simulink model "ME416_Autonomy_Model_Rollback2"  (R2025b)
settings: Solver=FixedStepAuto  StartTime=0.0  StopTime=240  RelTol=1e-3  EnableMultiTasking=on
PreLoadFcn:
  | driveparam
values from neighbouring files (symbols this model uses):
  alpha_w = 0.7    [driveparam.m]
  beta = Ts / (Ts + tau)    (= 0.166666666667)    [driveparam.m]
  enable_cmd = 1    [driveparam.m]
  estop_cmd = 0    [driveparam.m]
  K_lqr_w = dlqr(Ad_w, Bd_w, Qw, Rw)    [driveparam.m]
  L = 0.15    [driveparam.m]
  N = 4400    [driveparam.m]
  Nbar_lqr_w = (1 - Ad_w)/Bd_w + K_lqr_w    [driveparam.m]
  r = 0.03    [driveparam.m]
  Ts = 0.01    [driveparam.m]
  v_ref_cmd = 0    [driveparam.m]
  w_ref_cmd = 0.1    [driveparam.m]
undefined symbols (not defined in the file or in its folder): DiscIntNeverNeededParam, dspblkCoreblockFVToolHelper, gcbh
libraries: raspberrypiBasiclib x22, simulink x21, raspberrypiCommlib x19, slpidlib x2
(part 1 of 3)
settings Model: ExtModeTrigDuration=2  Creator=madak  LastModifiedBy=madak
settings SolverCC: PositivePriorityOrder=on  AutoInsertRateTranBlk=on
settings OptimizationCC: EnhancedBackFolding=on  PassReuseOutputArgsAs=Individual arguments  ZeroExternalMemoryAtStartup=off  ZeroInternalMemoryAtStartup=off  MaxStackSize=200000  OptimizeBlockOrder=speed  DifferentSizesBufferReuse=on  OptimizationCustomize=off  EfficientTunableParamExpr=on
settings DebuggingCC: ParameterPrecisionLossMsg=none  ParameterTunabilityLossMsg=error
settings HardwareCC: ProdBitPerLong=64.0  ProdLargestAtomicInteger=LongLong  ProdLargestAtomicFloat=Double  ProdLongLongMode=on  ProdHWDeviceType=ARM Compatible->ARM Cortex-A (64-bit)
settings RTWCC: SystemTargetFile=ert.tlc  HardwareBoard=Raspberry Pi (64bit)  TLCOptions="-aInlineSetEventsForThisBaseRateFcn=TLC_FALSE -aSuppressMultiTaskScheduler=TLC_FALSE  -aRateBasedStepFcn=0"  TemplateMakefile=ert_default_tmf  Toolchain=GNU GCC Embedded Linux  BuildConfiguration=Faster Runs  GPUComputeCapability=3.5  Description=Embedded Coder
settings CodeAppCC: ForceParamTrailComments=on  IgnoreCustomStorageClasses=off  OperatorAnnotations=on  SimulinkDataObjDesc=on  SFDataObjDesc=on  InsertBlockDesc=on
settings ERTTargetCC: ExtModeTransport=2.0  ExtModeStaticAlloc=on  ExtModeMexFile=ext_xcp  ExtModeIntrfLevel=Level2 - Open  InlinedParameterPlacement=Hierarchical  CodeReplacementLibrary=ARM Cortex-A CMSIS  SupportContinuousTime=on  SupportVariableSizeSignals=on

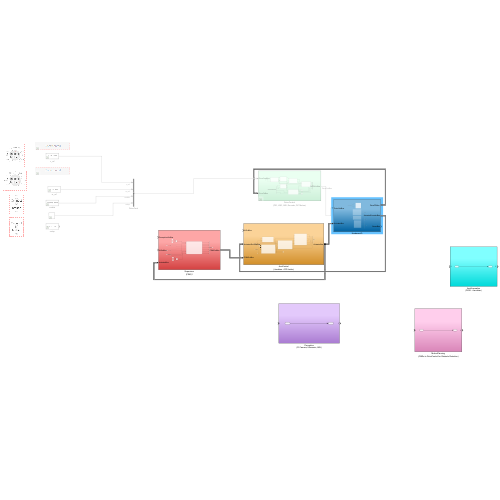
[thumbnail: Simulink's stored preview of the top-level diagram]
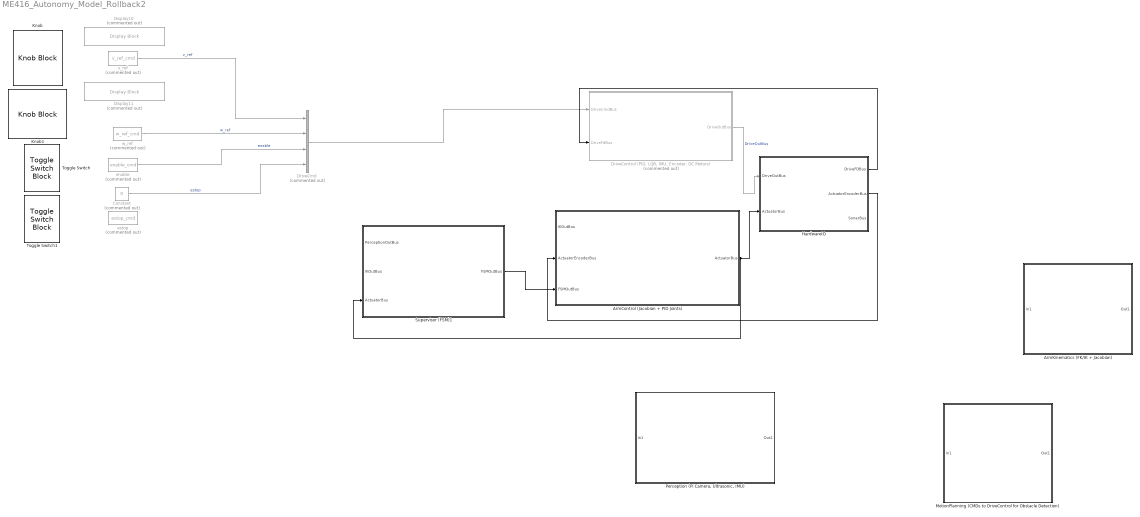
== system ME416_Autonomy_Model_Rollback2 ==
  ArmControl (Jacobian + PID Joints) : Subsystem
  ArmKinematics (FK/IK + Jacobian) : Subsystem
  Constant : Constant  Commented=on  Value=0
  Display10 : DisplayBlock  Commented=on  LabelPosition=Hide  Transparency=1  GridColor=[0.502, 0.502, 0.502]
  Display11 : DisplayBlock  Commented=on  LabelPosition=Hide  Transparency=1  GridColor=[0.502, 0.502, 0.502]
  DriveCmd : BusCreator  Commented=on  Inputs=4
  "DriveControl (PID, LQR, IMU, Encoder, DC Motors)" : Subsystem  Commented=on
  HardwareIO : Subsystem
  Knob : KnobBlock  ScaleMin=-0.5  ScaleMax=0.5  TickInterval=0.1
  Knob1 : KnobBlock  ScaleMin=-1  ScaleMax=1
  MotionPlanning (CMDs to DriveControl for Obstacle Detection) : Subsystem
  "Perception (Pi Camera, Ultrasonic, IMU)" : Subsystem
  Supervisor (FSM)1 : Subsystem
  Toggle Switch : ToggleSwitchBlock
  Toggle Switch1 : ToggleSwitchBlock
  enable : Constant  Commented=on  Value=enable_cmd
  estop : Constant  Commented=on  Value=estop_cmd  OutDataTypeStr=boolean
  v_ref : Constant  Commented=on  Value=v_ref_cmd
  w_ref : Constant  Commented=on  Value=w_ref_cmd
  wires:
  DriveCmd/1 -> "DriveControl (PID, LQR, IMU, Encoder, DC Motors)"/1(DriveCmdBus)
  "DriveControl (PID, LQR, IMU, Encoder, DC Motors)"/1(DriveOutBus) -> HardwareIO/1(DriveOutBus)  "DriveOutBus"
  v_ref/1 -> DriveCmd/1  "v_ref"
  w_ref/1 -> DriveCmd/2  "w_ref"
  enable/1 -> DriveCmd/3  "enable"
  Constant/1 -> DriveCmd/4  "estop"
  HardwareIO/1("DriveFDBus ") -> "DriveControl (PID, LQR, IMU, Encoder, DC Motors)"/2(DriveFdBus)
  ArmControl (Jacobian + PID Joints)/1(ActuatorBus) -> Supervisor (FSM)1/3(ActuatorBus), HardwareIO/2(ActuatorBus)
  HardwareIO/2(ActuatorEncoderBus) -> ArmControl (Jacobian + PID Joints)/2(ActuatorEncoderBus)
  Supervisor (FSM)1/1(FSMOutBus) -> ArmControl (Jacobian + PID Joints)/3(FSMOutBus)

== system ME416_Autonomy_Model_Rollback2/ArmControl (Jacobian + PID Joints) ==
  IKOutBus : Inport
  ActuatorEncoderBus : Inport  Port=2
  FSMOutBus : Inport  Port=3
  ActuatorMapping : Subsystem
  Bus Creator : BusCreator  Inputs=8
  Bus Selector : BusSelector  OutputSignals=imu2_yaw_rate,imu3_pitch
  Bus Selector1 : BusSelector  Commented=on  OutputSignals=is_poweron,is_post,is_search,is_chase,is_compute,is_actuate,drive_stop_cmd
  Constant : Constant
  Constant1 : Constant  Value=0
  HoldAndStabilize : Subsystem
  JointController : Subsystem
  ReferenceManager : Subsystem
  Scope : Scope  NumInputPorts=2
      settings: ActiveDisplayYMinimum=-0.12499999999999997  ActiveDisplayYMaximum=1.125  DataLoggingVariableName=ScopeData2
  ActuatorBus : Outport
  wires:
  ActuatorEncoderBus/1 -> Bus Selector/1
  Bus Creator/1 -> ActuatorBus/1
  JointController/3(post_done) -> Bus Creator/7  "post_done"
  JointController/4(actuation_done) -> Bus Creator/8  "actuation_done"
  HoldAndStabilize/1(femur_hold_cmd) -> JointController/3(femur_hold_cmd)
  ReferenceManager/1(base_servo_stabilize_enable) -> JointController/5(base_servo_stabilize_enable)
  ReferenceManager/2(femur_ref) -> JointController/1(femur_ref)
  ReferenceManager/3(stepper_mode) -> ActuatorMapping/2(stepper_mode)
  ReferenceManager/4(gripper_ref) -> ActuatorMapping/4(gripper_ref)
  ReferenceManager/5(base_servo_post_enable) -> Scope/1, JointController/6(base_servo_post_enable)  "base_servo_post_enable"
  ReferenceManager/6(base_servo_actuate_enable) -> Scope/2, JointController/7(base_servo_actuate_enable)  "base_servo_actuate_enable"
  JointController/1(femur_actuator_cmd) -> ActuatorMapping/3(femur_actuator_cmd)
  ActuatorMapping/5(femur_servo_pwm) -> Bus Creator/5  "femur_servo_pwm"
  ActuatorMapping/2(stepper_enable) -> Bus Creator/2  "stepper_enable"
  ActuatorMapping/1(base_servo_pwm) -> Bus Creator/1  "base_servo_pwm"
  JointController/2(base_servo_cmd) -> ActuatorMapping/1(base_servo_cmd)
  ActuatorMapping/3(stepper_dir) -> Bus Creator/3  "stepper_dir"
  ActuatorMapping/6(gripper_servo_pwm) -> Bus Creator/6  "gripper_servo_pwm"
  ActuatorMapping/4(stepper_step) -> Bus Creator/4  "stepper_step"
  Bus Selector/1 -> JointController/4(imu2_yaw_rate)  "<imu2_yaw_rate>"
  Bus Selector/2 -> JointController/2(imu3_pitch), HoldAndStabilize/2(<imu3_pitch>)  "<imu3_pitch>"
  FSMOutBus/1 -> Bus Selector1/1
  Constant1/1 -> ReferenceManager/5(is_compute), ReferenceManager/4(is_chase), ReferenceManager/3(is_search), ReferenceManager/1(is_poweron), HoldAndStabilize/1(is_poweron)
  Constant/1 -> ReferenceManager/2(is_post)

== system ME416_Autonomy_Model_Rollback2/ArmKinematics (FK//IK + Jacobian) ==
  In1 : Inport
  Out1 : Outport
  wires:
  In1/1 -> Out1/1

== system ME416_Autonomy_Model_Rollback2/DriveControl (PID, LQR, IMU, Encoder, DC Motors) ==
  DriveCmdBus : Inport
  DriveFdBus : Inport  Port=2
  Bus Creator : BusCreator  Inputs=8
  BusSel_DriveCmd : BusSelector  Commented=on  OutputSignals=v_ref,w_ref,enable,estop
  BusSel_DriveFd : BusSelector  OutputSignals=enc_left_ticks,enc_right_ticks,imu1_yaw_rate,imu1_pitch
  CommandSafety : Subsystem
  DifferentialDrive : Subsystem
  EncoderSpeed : Subsystem
  OutputSafety : Subsystem
  Scope : Scope  NumInputPorts=2
      settings: ActiveDisplayYMinimum=-1  ActiveDisplayYMaximum=1
  Scope1 : Scope  NumInputPorts=2
      settings: ActiveDisplayYMinimum=-1  ActiveDisplayYMaximum=1
  StateEstimate : Subsystem
  WheelPI : Subsystem
  DriveOutBus : Outport
  wires:
  DriveCmdBus/1 -> BusSel_DriveCmd/1
  StateEstimate/4(w_meas) -> OutputSafety/6(w_meas)
  DriveFdBus/1 -> BusSel_DriveFd/1
  StateEstimate/6(x_hat) -> Bus Creator/7  "x_hat"
  BusSel_DriveCmd/1 -> CommandSafety/1(v_ref)  "<v_ref>"
  CommandSafety/2(w_cmd) -> DifferentialDrive/2(w_cmd)
  BusSel_DriveCmd/2 -> CommandSafety/2(w_ref)  "<w_ref>"
  BusSel_DriveCmd/4 -> CommandSafety/4(estop)  "<estop>"
  BusSel_DriveCmd/3 -> CommandSafety/3(enable)  "<enable>"
  CommandSafety/1(v_cmd) -> DifferentialDrive/1(v_cmd)
  CommandSafety/3(drive_enable) -> OutputSafety/3(drive_enable)
  CommandSafety/4(estop_active) -> OutputSafety/4(estop_active)
  StateEstimate/3(v_meas) -> OutputSafety/5(v_meas)
  BusSel_DriveFd/1 -> EncoderSpeed/1(enc_left_ticks)  "<enc_left_ticks>"
  BusSel_DriveFd/2 -> EncoderSpeed/2(enc_right_ticks)  "<enc_right_ticks>"
  BusSel_DriveFd/3 -> StateEstimate/3(imu_yaw_rate)  "<imu1_yaw_rate>"
  BusSel_DriveFd/4 -> StateEstimate/4(imu_pitch)  "<imu1_pitch>"
  DifferentialDrive/1(omega_left_ref) -> WheelPI/1(omega_left_ref)
  DifferentialDrive/2(omega_right_ref) -> WheelPI/2(omega_right_ref)
  EncoderSpeed/1(omega_left_meas) -> StateEstimate/1(omega_left_meas), WheelPI/3(omega_left_meas)
  EncoderSpeed/2(omega_right_meas) -> WheelPI/4(omega_right_meas), StateEstimate/2(omega_right_meas)
  WheelPI/1(u_left_raw) -> OutputSafety/1(u_left_raw)
  WheelPI/2(u_right_raw) -> OutputSafety/2(u_right_raw)
  Bus Creator/1 -> DriveOutBus/1
  StateEstimate/9(y_dot) -> Scope1/2
  StateEstimate/1(yaw_rate_meas) -> Scope/1
  StateEstimate/2(pitch_meas) -> Scope/2
  StateEstimate/5(theta_hat) -> Bus Creator/6  "theta_hat"
  StateEstimate/7(x_dot) -> Scope1/1
  StateEstimate/8(y_hat) -> Bus Creator/8  "y_hat"
  OutputSafety/1(u_left) -> Bus Creator/1  "u_left"
  OutputSafety/2(u_right) -> Bus Creator/2  "u_right"
  OutputSafety/3(v_meas_out) -> Bus Creator/3  "v_meas_out"
  OutputSafety/4(w_meas_out) -> Bus Creator/4  "w_meas_out"
  OutputSafety/5(estop_active_out) -> Bus Creator/5  "estop_active_out"

== system ME416_Autonomy_Model_Rollback2/HardwareIO ==
  DriveOutBus : Inport
  ActuatorBus : Inport  Port=2
  ArmActuators_System : Subsystem
  Bus Creator : BusCreator  Inputs=8
  Bus Creator1 : BusCreator  Inputs=3
  Bus Creator2 : BusCreator  Inputs=12
  Bus Selector : BusSelector  OutputSignals=base_servo_pwm,femur_servo_pwm,stepper_enable,stepper_dir,stepper_step,gripper_servo_pwm
  Encoder_System : Subsystem  Commented=on
  IMU_System : Subsystem  Commented=on
  Ultrasonic_System : Subsystem  Commented=on
  "DriveFDBus " : Outport
  ActuatorEncoderBus : Outport  Port=2
  SonarBus : Outport  Port=3
  wires:
  Ultrasonic_System/3(ultrasonic_front) -> Bus Creator1/3  "ultrasonic_front"
  Bus Creator2/1 -> ActuatorEncoderBus/1
  Bus Creator/1 -> "DriveFDBus "/1
  IMU_System/2(imu1_ay) -> Bus Creator/4  "imu1_y"
  Bus Creator1/1 -> SonarBus/1
  Encoder_System/2(enc_right_ticks) -> Bus Creator/2  "enc_right_ticks"
  IMU_System/9(imu2_az) -> Bus Creator2/3  "imu2_az"
  IMU_System/16(imu3_pitch) -> Bus Creator2/10  "imu3_pitch"
  Bus Selector/1 -> ArmActuators_System/1(base_servo_cmd)  "<base_servo_pwm>"
  Bus Selector/6 -> ArmActuators_System/6(gripper_cmd)  "<gripper_servo_pwm>"
  IMU_System/11(imu2_roll) -> Bus Creator2/5  "imu2_roll"
  IMU_System/3(imu1_az) -> Bus Creator/5  "imu1_az"
  IMU_System/18(imu3_yaw_rate) -> Bus Creator2/12  "imu3_yaw_rate"
  IMU_System/10(imu2_pitch) -> Bus Creator2/4  "imu2_pitch"
  IMU_System/8(imu2_ay) -> Bus Creator2/2  "imu2_ay"
  IMU_System/1(imu1_ax) -> Bus Creator/3  "imu1_ax"
  Ultrasonic_System/2(ultrasonic_right) -> Bus Creator1/2  "ultrasonic_right"
  Bus Selector/2 -> ArmActuators_System/2(femur_servo_cmd)  "<femur_servo_pwm>"
  IMU_System/7(imu2_ax) -> Bus Creator2/1  "imu2_ax"
  IMU_System/12(imu2_yaw_rate) -> Bus Creator2/6  "imu2_yaw_rate"
  IMU_System/5(imu1_roll) -> Bus Creator/7  "imu1_roll"
  Bus Selector/3 -> ArmActuators_System/3(stepper_enable)  "<stepper_enable>"
  Encoder_System/1(enc_left_ticks) -> Bus Creator/1  "enc_left_ticks"
  Ultrasonic_System/1(ultrasonic_left) -> Bus Creator1/1  "ultrasonic_left"
  IMU_System/15(imu3_az) -> Bus Creator2/9  "imu3_az"
  DriveOutBus/1 -> Encoder_System/1(DriveOutBus)
  Bus Selector/5 -> ArmActuators_System/5(stepper_step_cmd)  "<stepper_step>"
  IMU_System/6(imu1_yaw_rate) -> Bus Creator/8  "imu1_yaw_rate"
  IMU_System/17(imu3_roll) -> Bus Creator2/11  "imu3_roll"
  Bus Selector/4 -> ArmActuators_System/4(stepper_dir_cmd)  "<stepper_dir>"
  ActuatorBus/1 -> Bus Selector/1
  IMU_System/4(imu1_pitch) -> Bus Creator/6  "imu1_pitch"
  IMU_System/13(imu3_ax) -> Bus Creator2/7  "imu3_ax"
  IMU_System/14(imu3_ay) -> Bus Creator2/8  "imu3_ay"

== system ME416_Autonomy_Model_Rollback2/MotionPlanning (CMDs to DriveControl for Obstacle Detection) ==
  In1 : Inport
  Out1 : Outport
  wires:
  In1/1 -> Out1/1

== system ME416_Autonomy_Model_Rollback2/Perception (Pi Camera, Ultrasonic, IMU) ==
  In1 : Inport
  Out1 : Outport
  wires:
  In1/1 -> Out1/1

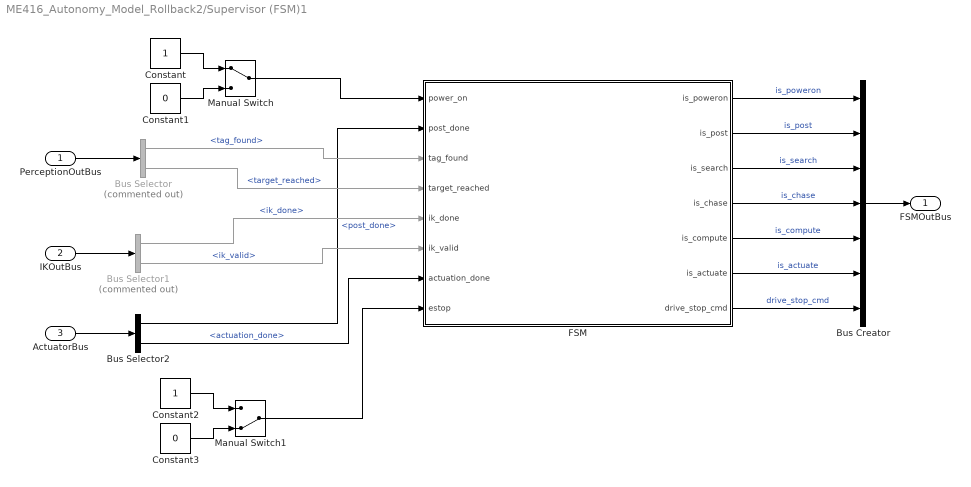
== system ME416_Autonomy_Model_Rollback2/Supervisor (FSM)1 ==
  PerceptionOutBus : Inport
  IKOutBus : Inport  Port=2
  ActuatorBus : Inport  Port=3
  Bus Creator : BusCreator  Inputs=7
  Bus Selector : BusSelector  Commented=on  OutputSignals=tag_found,target_reached
  Bus Selector1 : BusSelector  Commented=on  OutputSignals=ik_done,ik_valid
  Bus Selector2 : BusSelector  OutputSignals=post_done,actuation_done
  Constant : Constant
  Constant1 : Constant  Value=0
  Constant2 : Constant
  Constant3 : Constant  Value=0
  FSM : Stateflow chart  TreatAsAtomicUnit=on
  Manual Switch : ManualSwitch
  Manual Switch1 : ManualSwitch  CurrentSetting=0
  FSMOutBus : Outport
  wires:
  Manual Switch/1 -> FSM/1(power_on)
  Bus Selector2/1 -> FSM/2(post_done)  "<post_done>"
  Bus Selector2/2 -> FSM/7(actuation_done)  "<actuation_done>"
  Bus Selector/2 -> FSM/4(target_reached)  "<target_reached>"
  Bus Selector1/1 -> FSM/5(ik_done)  "<ik_done>"
  Manual Switch1/1 -> FSM/8(estop)
  FSM/1(is_poweron) -> Bus Creator/1  "is_poweron"
  FSM/2(is_post) -> Bus Creator/2  "is_post"
  FSM/5(is_compute) -> Bus Creator/5  "is_compute"
  FSM/3(is_search) -> Bus Creator/3  "is_search"
  FSM/4(is_chase) -> Bus Creator/4  "is_chase"
  FSM/6(is_actuate) -> Bus Creator/6  "is_actuate"
  FSM/7(drive_stop_cmd) -> Bus Creator/7  "drive_stop_cmd"
  Bus Creator/1 -> FSMOutBus/1
  PerceptionOutBus/1 -> Bus Selector/1
  Bus Selector/1 -> FSM/3(tag_found)  "<tag_found>"
  IKOutBus/1 -> Bus Selector1/1
  Bus Selector1/2 -> FSM/6(ik_valid)  "<ik_valid>"
  ActuatorBus/1 -> Bus Selector2/1
  Constant/1 -> Manual Switch/1
  Constant1/1 -> Manual Switch/2
  Constant2/1 -> Manual Switch1/1
  Constant3/1 -> Manual Switch1/2

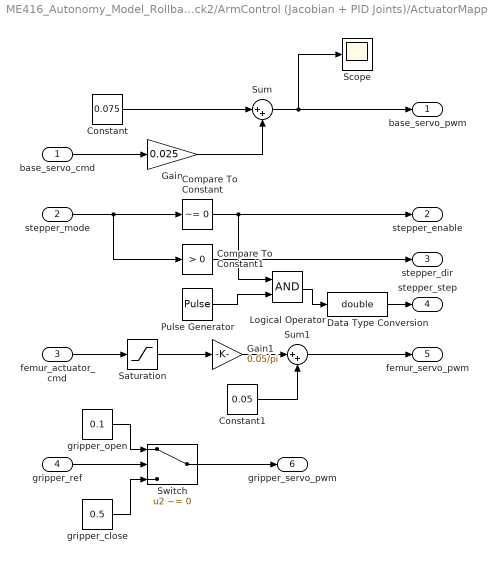
== system ME416_Autonomy_Model_Rollback2/ArmControl (Jacobian + PID Joints)/ActuatorMapping ==
  base_servo_cmd : Inport
  stepper_mode : Inport  Port=2
  femur_actuator_cmd : Inport  Port=3
  gripper_ref : Inport  Port=4
  Compare To Constant : simulink/Logic and Bit Operations/Compare To Constant  relop=~=  const=0  OutDataTypeStr=boolean
  Compare To Constant1 : simulink/Logic and Bit Operations/Compare To Constant  relop=>  const=0  OutDataTypeStr=boolean
  Constant : Constant  Value=0.075
  Constant1 : Constant  Value=0.05
  Data Type Conversion : DataTypeConversion  OutDataTypeStr=double  SaturateOnIntegerOverflow=off  RndMeth=Floor
  Gain : Gain  Gain=0.025
  Gain1 : Gain  Gain=0.05/pi
  Logical Operator : Logic  AllPortsSameDT=off  OutDataTypeStr=boolean
  Pulse Generator : DiscretePulseGenerator  PulseType=Time based  Period=10  PulseWidth=5
  Saturation : Saturate  UpperLimit=pi  LowerLimit=0
  Scope : Scope
      settings: DataLoggingVariableName=ScopeData3
  Sum : Sum  Inputs=|++
  Sum1 : Sum  Inputs=|++
  Switch : Switch  Criteria=u2 ~= 0  SaturateOnIntegerOverflow=off  InputSameDT=off
  gripper_close : Constant  Value=0.5
  gripper_open : Constant  Value=0.1
  base_servo_pwm : Outport
  stepper_enable : Outport  Port=2
  stepper_dir : Outport  Port=3
  stepper_step : Outport  Port=4
  femur_servo_pwm : Outport  Port=5
  gripper_servo_pwm : Outport  Port=6
  wires:
  Sum1/1 -> femur_servo_pwm/1
  stepper_mode/1 -> Compare To Constant1/1, Compare To Constant/1
  femur_actuator_cmd/1 -> Saturation/1
  Saturation/1 -> Gain1/1
  base_servo_cmd/1 -> Gain/1
  Gain/1 -> Sum/2
  Constant/1 -> Sum/1
  Sum/1 -> Scope/1, base_servo_pwm/1
  Gain1/1 -> Sum1/1
  Constant1/1 -> Sum1/2
  gripper_open/1 -> Switch/1
  gripper_close/1 -> Switch/3
  gripper_ref/1 -> Switch/2
  Switch/1 -> gripper_servo_pwm/1
  Compare To Constant/1 -> stepper_enable/1, Logical Operator/1
  Compare To Constant1/1 -> stepper_dir/1
  Pulse Generator/1 -> Logical Operator/2
  Data Type Conversion/1 -> stepper_step/1
  Logical Operator/1 -> Data Type Conversion/1

== system ME416_Autonomy_Model_Rollback2/ArmControl (Jacobian + PID Joints)/HoldAndStabilize ==
  is_poweron : Inport
  <imu3_pitch> : Inport  Port=2
  Add : Sum
  Constant : Constant  Value=0
  Kd_pitch_rate : Gain  Gain=-0.3
  Kp_pitch : Gain  Gain=2
  Saturation : Saturate  UpperLimit=1  LowerLimit=-1
  compute_pitch_error : Sum  Inputs=|+-
  latch_pitch_ref : Subsystem  TreatAsAtomicUnit=on
  poweron_detect_rise : simulink/Logic and Bit Operations/Detect Rise Positive  vinit=0  OutDataTypeStr=boolean
  femur_hold_cmd : Outport
  wires:
  Add/1 -> Saturation/1  "u_hold_raw"
  <imu3_pitch>/1 -> latch_pitch_ref/1(imu3_pitch), compute_pitch_error/2
  is_poweron/1 -> poweron_detect_rise/1
  latch_pitch_ref/1(pitch_ref) -> compute_pitch_error/1
  Kp_pitch/1 -> Add/1
  Kd_pitch_rate/1 -> Add/2
  poweron_detect_rise/1 -> latch_pitch_ref/Trigger
  compute_pitch_error/1 -> Kp_pitch/1  "pitch_error"
  Constant/1 -> Kd_pitch_rate/1
  Saturation/1 -> femur_hold_cmd/1  "femur_hold_cmd"

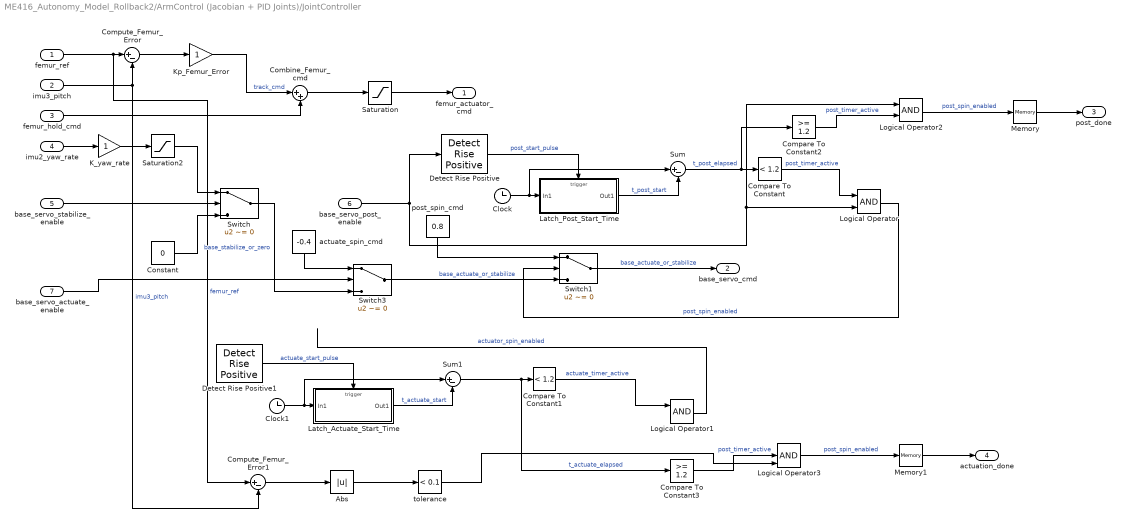
== system ME416_Autonomy_Model_Rollback2/ArmControl (Jacobian + PID Joints)/JointController ==
  femur_ref : Inport
  imu3_pitch : Inport  Port=2
  femur_hold_cmd : Inport  Port=3
  imu2_yaw_rate : Inport  Port=4
  base_servo_stabilize_enable : Inport  Port=5
  base_servo_post_enable : Inport  Port=6
  base_servo_actuate_enable : Inport  Port=7
  Abs : Abs  SaturateOnIntegerOverflow=off
  Clock : Clock
  Clock1 : Clock
  Combine_Femur_cmd : Sum  Inputs=|++
  Compare To Constant : simulink/Logic and Bit Operations/Compare To Constant  relop=<  const=1.2  OutDataTypeStr=boolean
  Compare To Constant1 : simulink/Logic and Bit Operations/Compare To Constant  relop=<  const=1.2  OutDataTypeStr=boolean
  Compare To Constant2 : simulink/Logic and Bit Operations/Compare To Constant  relop=>=  const=1.2  OutDataTypeStr=boolean
  Compare To Constant3 : simulink/Logic and Bit Operations/Compare To Constant  relop=>=  const=1.2  OutDataTypeStr=boolean
  Compute_Femur_Error : Sum  Inputs=|+-
  Compute_Femur_Error1 : Sum  Inputs=|+-
  Constant : Constant  Value=0
  Detect Rise Positive : simulink/Logic and Bit Operations/Detect Rise Positive  vinit=0  OutDataTypeStr=boolean
  Detect Rise Positive1 : simulink/Logic and Bit Operations/Detect Rise Positive  vinit=0  OutDataTypeStr=boolean
  K_yaw_rate : Gain
  Kp_Femur_Error : Gain
  Latch_Actuate_Start_Time : Subsystem  TreatAsAtomicUnit=on
  Latch_Post_Start_Time : Subsystem  TreatAsAtomicUnit=on
  Logical Operator : Logic  AllPortsSameDT=off  OutDataTypeStr=boolean
  Logical Operator1 : Logic  AllPortsSameDT=off  OutDataTypeStr=boolean
  Logical Operator2 : Logic  AllPortsSameDT=off  OutDataTypeStr=boolean
  Logical Operator3 : Logic  Inputs=3  AllPortsSameDT=off  OutDataTypeStr=boolean
  Memory : Memory
  Memory1 : Memory
  Saturation : Saturate  UpperLimit=1  LowerLimit=-1
  Saturation2 : Saturate  UpperLimit=1  LowerLimit=-1
  Sum : Sum  Inputs=|+-
  Sum1 : Sum  Inputs=|+-
  Switch : Switch  Criteria=u2 ~= 0  SaturateOnIntegerOverflow=off  InputSameDT=off
  Switch1 : Switch  Criteria=u2 ~= 0  SaturateOnIntegerOverflow=off  InputSameDT=off
  Switch3 : Switch  Criteria=u2 ~= 0  SaturateOnIntegerOverflow=off  InputSameDT=off
  actuate_spin_cmd : Constant  Value=-0.4
  post_spin_cmd : Constant  Value=0.8
  tolerance : simulink/Logic and Bit Operations/Compare To Constant  relop=<  const=0.1  OutDataTypeStr=boolean
  femur_actuator_cmd : Outport
  base_servo_cmd : Outport  Port=2
  post_done : Outport  Port=3
  actuation_done : Outport  Port=4
  wires:
  femur_ref/1 -> Compute_Femur_Error1/1, Compute_Femur_Error/1  "femur_ref"
  imu3_pitch/1 -> Compute_Femur_Error1/2, Compute_Femur_Error/2  "imu3_pitch"
  Compute_Femur_Error/1 -> Kp_Femur_Error/1
  Combine_Femur_cmd/1 -> Saturation/1
  Saturation/1 -> femur_actuator_cmd/1
  Kp_Femur_Error/1 -> Combine_Femur_cmd/1  "track_cmd"
  femur_hold_cmd/1 -> Combine_Femur_cmd/2
  imu2_yaw_rate/1 -> K_yaw_rate/1
  K_yaw_rate/1 -> Saturation2/1
  Constant/1 -> Switch/3
  base_servo_stabilize_enable/1 -> Switch/2
  Saturation2/1 -> Switch/1
  Switch/1 -> Switch3/3  "base_stabilize_or_zero"
  Switch3/1 -> Switch1/3  "base_actuate_or_stabilize"
  actuate_spin_cmd/1 -> Switch3/1
  post_spin_cmd/1 -> Switch1/1
  base_servo_post_enable/1 -> Logical Operator/2, Logical Operator2/1, Detect Rise Positive/1
  Detect Rise Positive/1 -> Latch_Post_Start_Time/Trigger  "post_start_pulse"
  Clock/1 -> Sum/1, Latch_Post_Start_Time/1(In1)
  Latch_Post_Start_Time/1(Out1) -> Sum/2  "t_post_start"
  Sum/1 -> Compare To Constant/1, Compare To Constant2/1  "t_post_elapsed"
  Compare To Constant/1 -> Logical Operator/1  "post_timer_active"
  Logical Operator/1 -> Switch1/2  "post_spin_enabled"
  Sum1/1 -> Compare To Constant3/1, Compare To Constant1/1  "t_actuate_elapsed"
  Detect Rise Positive1/1 -> Latch_Actuate_Start_Time/Trigger  "actuate_start_pulse"
  Clock1/1 -> Sum1/1, Latch_Actuate_Start_Time/1(In1)
  Compare To Constant1/1 -> Logical Operator1/1  "actuate_timer_active"
  Latch_Actuate_Start_Time/1(Out1) -> Sum1/2  "t_actuate_start"
  Logical Operator1/1 -> ?  "actuator_spin_enabled"
  Compare To Constant2/1 -> Logical Operator2/2  "post_timer_active"
  Logical Operator2/1 -> Memory/1  "post_spin_enabled"
  Compare To Constant3/1 -> Logical Operator3/2  "post_timer_active"
  ? -> Logical Operator3/1, Logical Operator1/2, Detect Rise Positive1/1
  Logical Operator3/1 -> Memory1/1  "post_spin_enabled"
  Compute_Femur_Error1/1 -> Abs/1
  Abs/1 -> tolerance/1
  tolerance/1 -> Logical Operator3/3
  Memory/1 -> post_done/1
  Memory1/1 -> actuation_done/1
  Switch1/1 -> base_servo_cmd/1  "base_actuate_or_stabilize"
  base_servo_actuate_enable/1 -> Switch3/2

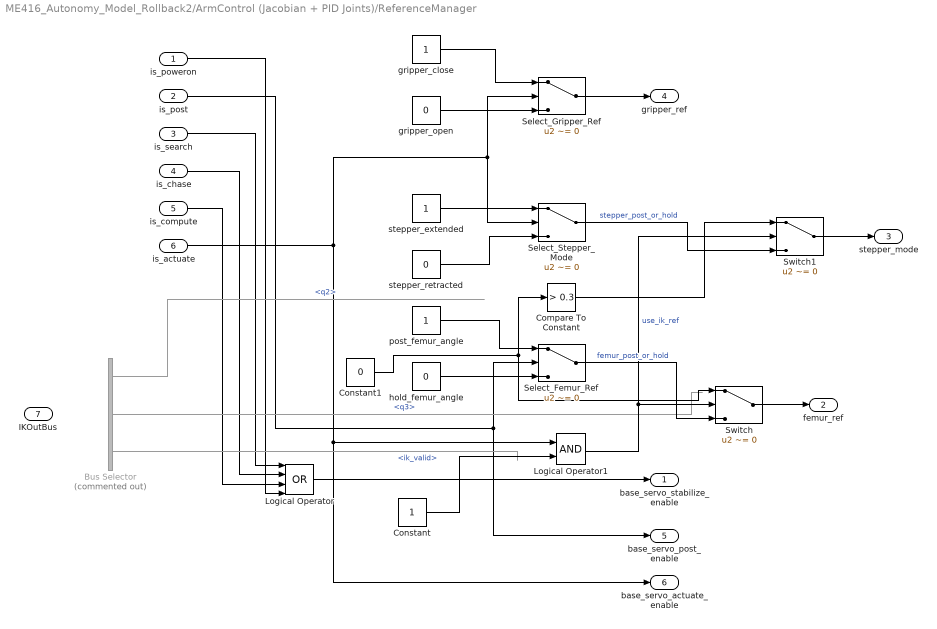
== system ME416_Autonomy_Model_Rollback2/ArmControl (Jacobian + PID Joints)/ReferenceManager ==
  is_poweron : Inport
  is_post : Inport  Port=2
  is_search : Inport  Port=3
  is_chase : Inport  Port=4
  is_compute : Inport  Port=5
  is_actuate : Inport  Port=6
  IKOutBus : Inport  Port=7
  Bus Selector : BusSelector  Commented=on  OutputSignals=q2,q3,ik_valid
  Compare To Constant : simulink/Logic and Bit Operations/Compare To Constant  relop=>  const=0.3  OutDataTypeStr=boolean
  Constant : Constant
  Constant1 : Constant  Value=0
  Logical Operator : Logic  Operator=OR  Inputs=4  AllPortsSameDT=off  OutDataTypeStr=boolean
  Logical Operator1 : Logic  AllPortsSameDT=off  OutDataTypeStr=boolean
  Select_Femur_Ref : Switch  Criteria=u2 ~= 0  SaturateOnIntegerOverflow=off  InputSameDT=off
  Select_Gripper_Ref : Switch  Criteria=u2 ~= 0  SaturateOnIntegerOverflow=off  InputSameDT=off
  Select_Stepper_Mode : Switch  Criteria=u2 ~= 0  SaturateOnIntegerOverflow=off  InputSameDT=off
  Switch : Switch  Criteria=u2 ~= 0  SaturateOnIntegerOverflow=off  InputSameDT=off
  Switch1 : Switch  Criteria=u2 ~= 0  SaturateOnIntegerOverflow=off  InputSameDT=off
  gripper_close : Constant
  gripper_open : Constant  Value=0
  hold_femur_angle : Constant  Value=0
  post_femur_angle : Constant
  stepper_extended : Constant
  stepper_retracted : Constant  Value=0
  base_servo_stabilize_enable : Outport
  femur_ref : Outport  Port=2
  stepper_mode : Outport  Port=3
  gripper_ref : Outport  Port=4
  base_servo_post_enable : Outport  Port=5
  base_servo_actuate_enable : Outport  Port=6
  wires:
  is_actuate/1 -> Select_Gripper_Ref/2, Select_Stepper_Mode/2, Logical Operator1/1, base_servo_actuate_enable/1
  gripper_close/1 -> Select_Gripper_Ref/1
  gripper_open/1 -> Select_Gripper_Ref/3
  is_post/1 -> base_servo_post_enable/1, Select_Femur_Ref/2
  stepper_extended/1 -> Select_Stepper_Mode/1
  stepper_retracted/1 -> Select_Stepper_Mode/3
  Select_Gripper_Ref/1 -> gripper_ref/1
  post_femur_angle/1 -> Select_Femur_Ref/1
  hold_femur_angle/1 -> Select_Femur_Ref/3
  Logical Operator/1 -> base_servo_stabilize_enable/1
  is_search/1 -> Logical Operator/1
  is_chase/1 -> Logical Operator/2
  is_compute/1 -> Logical Operator/3
  is_poweron/1 -> Logical Operator/4
  Bus Selector/3 -> ?  "<ik_valid>"
  Bus Selector/2 -> ?  "<q3>"
  Select_Femur_Ref/1 -> Switch/3  "femur_post_or_hold"
  Logical Operator1/1 -> Switch/2, Switch1/2  "use_ik_ref"
  Switch/1 -> femur_ref/1
  Switch1/1 -> stepper_mode/1
  Select_Stepper_Mode/1 -> Switch1/3  "stepper_post_or_hold"
  Compare To Constant/1 -> Switch1/1
  Bus Selector/1 -> ?  "<q2>"
  Constant/1 -> Logical Operator1/2
  Constant1/1 -> Switch/1, Compare To Constant/1

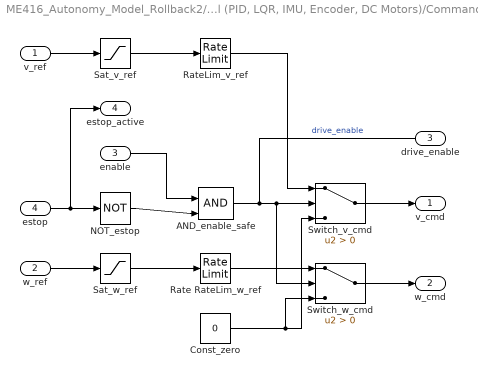
== system ME416_Autonomy_Model_Rollback2/DriveControl (PID, LQR, IMU, Encoder, DC Motors)/CommandSafety ==
  v_ref : Inport
  w_ref : Inport  Port=2
  enable : Inport  Port=3
  estop : Inport  Port=4
  AND_enable_safe : Logic  IconShape=distinctive  AllPortsSameDT=off  OutDataTypeStr=boolean
  Const_zero : Constant  Value=0
  NOT_estop : Logic  Operator=NOT  IconShape=distinctive  AllPortsSameDT=off  OutDataTypeStr=boolean
  Rate RateLim_w_ref : RateLimiter  SampleTimeMode=inherited
  RateLim_v_ref : RateLimiter  SampleTimeMode=inherited
  Sat_v_ref : Saturate  UpperLimit=0.6  LowerLimit=-0.6
  Sat_w_ref : Saturate  UpperLimit=1.5  LowerLimit=-1.5
  Switch_v_cmd : Switch  Criteria=u2 > Threshold  SaturateOnIntegerOverflow=off  InputSameDT=off
  Switch_w_cmd : Switch  Criteria=u2 > Threshold  SaturateOnIntegerOverflow=off  InputSameDT=off
  v_cmd : Outport
  w_cmd : Outport  Port=2
  drive_enable : Outport  Port=3
  estop_active : Outport  Port=4
  wires:
  v_ref/1 -> Sat_v_ref/1
  estop/1 -> NOT_estop/1, estop_active/1
  Sat_w_ref/1 -> Rate RateLim_w_ref/1
  w_ref/1 -> Sat_w_ref/1
  NOT_estop/1 -> AND_enable_safe/2
  Sat_v_ref/1 -> RateLim_v_ref/1
  enable/1 -> AND_enable_safe/1
  RateLim_v_ref/1 -> Switch_v_cmd/1
  AND_enable_safe/1 -> Switch_w_cmd/2, Switch_v_cmd/2, drive_enable/1  "drive_enable"
  Rate RateLim_w_ref/1 -> Switch_w_cmd/1
  Const_zero/1 -> Switch_v_cmd/3, Switch_w_cmd/3
  Switch_v_cmd/1 -> v_cmd/1
  Switch_w_cmd/1 -> w_cmd/1

== system ME416_Autonomy_Model_Rollback2/DriveControl (PID, LQR, IMU, Encoder, DC Motors)/DifferentialDrive ==
  v_cmd : Inport
  w_cmd : Inport  Port=2
  Gain_inv_r_left : Gain  Gain=1/r
  Product : Product
  Sum_v_left : Sum  Inputs=+-
  Sum_v_right : Sum
  gain_inv_r_right : Gain  Gain=1/r
  w_term : Constant  Value=L/2
  omega_left_ref : Outport
  omega_right_ref : Outport  Port=2
  wires:
  w_term/1 -> Product/1
  gain_inv_r_right/1 -> omega_right_ref/1
  w_cmd/1 -> Product/2
  v_cmd/1 -> Sum_v_right/1, Sum_v_left/1
  Sum_v_right/1 -> gain_inv_r_right/1  "v_right"
  Product/1 -> Sum_v_left/2, Sum_v_right/2
  Gain_inv_r_left/1 -> omega_left_ref/1
  Sum_v_left/1 -> Gain_inv_r_left/1  "v_left"

== system ME416_Autonomy_Model_Rollback2/DriveControl (PID, LQR, IMU, Encoder, DC Motors)/EncoderSpeed ==
  enc_left_ticks : Inport
  enc_right_ticks : Inport  Port=2
  DeltaTicks_left : Sum  Inputs=+-
  DeltaTicks_right : Sum  Inputs=+-
  Gain_rad2rads_left : Gain  Gain=1/Ts
  Gain_rad2rads_right : Gain  Gain=1/Ts
  Gain_ticks2rad_left : Gain  Gain=2*pi/N
  Gain_ticks2rad_right : Gain  Gain=2*pi/N
  LowPassFilter_left : DiscreteTransferFcn  LoadFcn=dspblkCoreblockFVToolHelper(gcbh,'load');  Numerator=[beta]  Denominator=[1 -(1 - beta)]  SampleTime=Ts
      settings: CopyFcn=dspblkCoreblockFVToolHelper(gcbh,'copy');  DeleteFcn=dspblkCoreblockFVToolHelper(gcbh,'close');  ModelCloseFcn=dspblkCoreblockFVToolHelper(gcbh,'close');  PreSaveFcn=dspblkCoreblockFVToolHelper(gcbh,'presave');  PostSaveFcn=dspblkCoreblockFVToolHelper(gcbh,'postsave');  CloseFcn=dspblkCoreblockFVToolHelper(gcbh,'close');
  LowPassFilter_right : DiscreteTransferFcn  Numerator=[beta]  Denominator=[1 -(1 - beta)]  SampleTime=Ts
  enc_left_UnitDelay : UnitDelay  SampleTime=-1  HasFrameUpgradeWarning=on
  enc_right_UnitDelay : UnitDelay  SampleTime=-1  HasFrameUpgradeWarning=on
  omega_left_meas : Outport
  omega_right_meas : Outport  Port=2
  wires:
  enc_left_ticks/1 -> DeltaTicks_left/1, enc_left_UnitDelay/1
  enc_right_ticks/1 -> DeltaTicks_right/1, enc_right_UnitDelay/1
  enc_right_UnitDelay/1 -> DeltaTicks_right/2
  enc_left_UnitDelay/1 -> DeltaTicks_left/2
  DeltaTicks_left/1 -> Gain_ticks2rad_left/1
  DeltaTicks_right/1 -> Gain_ticks2rad_right/1
  Gain_ticks2rad_right/1 -> Gain_rad2rads_right/1
  Gain_ticks2rad_left/1 -> Gain_rad2rads_left/1
  LowPassFilter_left/1 -> omega_right_meas/1
  Gain_rad2rads_right/1 -> LowPassFilter_left/1
  Gain_rad2rads_left/1 -> LowPassFilter_right/1
  LowPassFilter_right/1 -> omega_left_meas/1

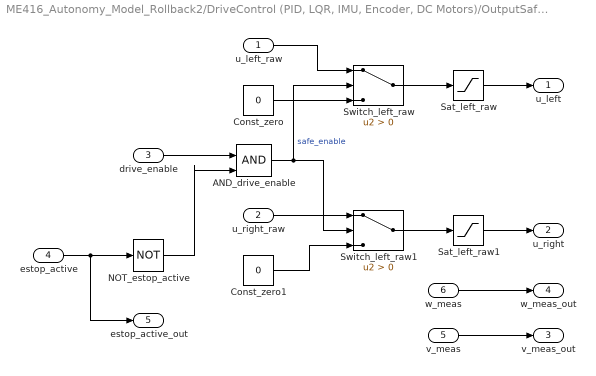
== system ME416_Autonomy_Model_Rollback2/DriveControl (PID, LQR, IMU, Encoder, DC Motors)/OutputSafety ==
  u_left_raw : Inport
  u_right_raw : Inport  Port=2
  drive_enable : Inport  Port=3
  estop_active : Inport  Port=4
  v_meas : Inport  Port=5
  w_meas : Inport  Port=6
  AND_drive_enable : Logic  IconShape=distinctive  AllPortsSameDT=off  OutDataTypeStr=boolean
  Const_zero : Constant  Value=0
  Const_zero1 : Constant  Value=0
  NOT_estop_active : Logic  Operator=NOT  IconShape=distinctive  AllPortsSameDT=off  OutDataTypeStr=boolean
  Sat_left_raw : Saturate  UpperLimit=1  LowerLimit=-1
  Sat_left_raw1 : Saturate  UpperLimit=1  LowerLimit=-1
  Switch_left_raw : Switch  Criteria=u2 > Threshold  SaturateOnIntegerOverflow=off  InputSameDT=off
  Switch_left_raw1 : Switch  Criteria=u2 > Threshold  SaturateOnIntegerOverflow=off  InputSameDT=off
  u_left : Outport
  u_right : Outport  Port=2
  v_meas_out : Outport  Port=3
  w_meas_out : Outport  Port=4
  estop_active_out : Outport  Port=5
  wires:
  u_left_raw/1 -> Switch_left_raw/1
  w_meas/1 -> w_meas_out/1
  v_meas/1 -> v_meas_out/1
  AND_drive_enable/1 -> Switch_left_raw1/2, Switch_left_raw/2  "safe_enable"
  estop_active/1 -> estop_active_out/1, NOT_estop_active/1
  drive_enable/1 -> AND_drive_enable/1
  NOT_estop_active/1 -> AND_drive_enable/2
  Const_zero/1 -> Switch_left_raw/3
  u_right_raw/1 -> Switch_left_raw1/1
  Const_zero1/1 -> Switch_left_raw1/3
  Switch_left_raw/1 -> Sat_left_raw/1
  Switch_left_raw1/1 -> Sat_left_raw1/1
  Sat_left_raw/1 -> u_left/1
  Sat_left_raw1/1 -> u_right/1

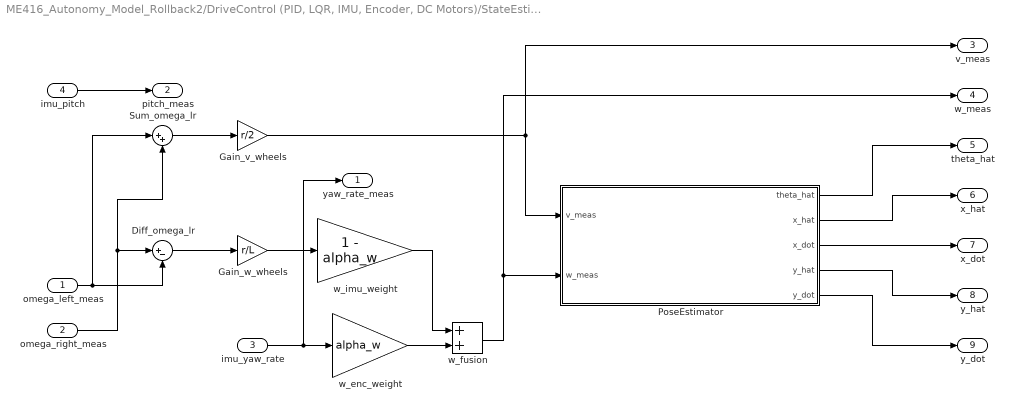
== system ME416_Autonomy_Model_Rollback2/DriveControl (PID, LQR, IMU, Encoder, DC Motors)/StateEstimate ==
  omega_left_meas : Inport
  omega_right_meas : Inport  Port=2
  imu_yaw_rate : Inport  Port=3
  imu_pitch : Inport  Port=4
  Diff_omega_lr : Sum  Inputs=|+-
  Gain_v_wheels : Gain  Gain=r/2
  Gain_w_wheels : Gain  Gain=r/L
  PoseEstimator : Subsystem
  Sum_omega_lr : Sum  Inputs=|++
  w_enc_weight : Gain  Gain=alpha_w
  w_fusion : Sum
  w_imu_weight : Gain  Gain=1 - alpha_w
  yaw_rate_meas : Outport
  pitch_meas : Outport  Port=2
  v_meas : Outport  Port=3
  w_meas : Outport  Port=4
  theta_hat : Outport  Port=5
  x_hat : Outport  Port=6
  x_dot : Outport  Port=7
  y_hat : Outport  Port=8
  y_dot : Outport  Port=9
  wires:
  omega_right_meas/1 -> Diff_omega_lr/1, Sum_omega_lr/2
  imu_pitch/1 -> pitch_meas/1
  imu_yaw_rate/1 -> yaw_rate_meas/1, w_enc_weight/1
  Gain_w_wheels/1 -> w_imu_weight/1
  omega_left_meas/1 -> Sum_omega_lr/1, Diff_omega_lr/2
  Sum_omega_lr/1 -> Gain_v_wheels/1
  Diff_omega_lr/1 -> Gain_w_wheels/1
  w_imu_weight/1 -> w_fusion/1
  w_enc_weight/1 -> w_fusion/2
  w_fusion/1 -> w_meas/1, PoseEstimator/2(w_meas)
  PoseEstimator/1(theta_hat) -> theta_hat/1
  PoseEstimator/2(x_hat) -> x_hat/1
  PoseEstimator/3(x_dot) -> x_dot/1
  PoseEstimator/4(y_hat) -> y_hat/1
  PoseEstimator/5(y_dot) -> y_dot/1
  Gain_v_wheels/1 -> PoseEstimator/1(v_meas), v_meas/1

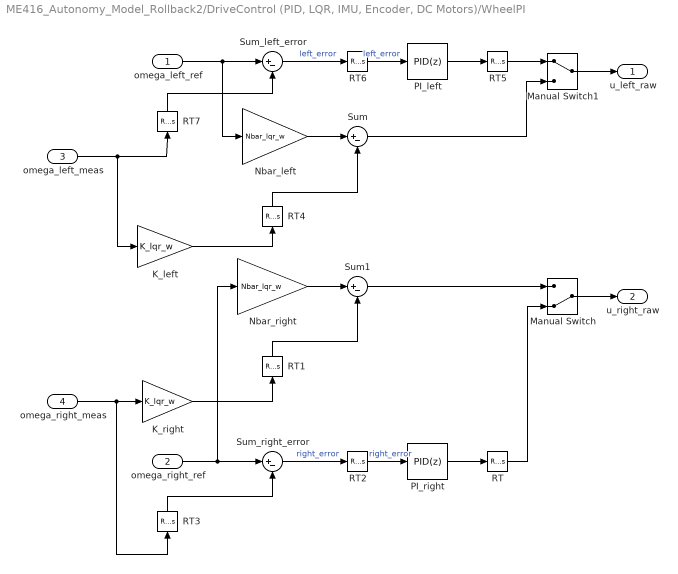
== system ME416_Autonomy_Model_Rollback2/DriveControl (PID, LQR, IMU, Encoder, DC Motors)/WheelPI ==
  omega_left_ref : Inport
  omega_right_ref : Inport  Port=2
  omega_left_meas : Inport  Port=3
  omega_right_meas : Inport  Port=4
  K_left : Gain  Gain=K_lqr_w
  K_right : Gain  Gain=K_lqr_w
  Manual Switch : ManualSwitch  CurrentSetting=0
  Manual Switch1 : ManualSwitch
  Nbar_left : Gain  Gain=Nbar_lqr_w
  Nbar_right : Gain  Gain=Nbar_lqr_w
  PI_left : slpidlib/PID Controller  Controller=PID  Form=Parallel  TimeDomain=Discrete-time  UseExternalTs=off  SampleTime=0.01  IntegratorMethod=Forward Euler  FilterMethod=Forward Euler  ControllerParametersSource=internal  P=0.02711  I=0.00415  UseKiTs=off  D=0  UseExternalDerivativeSource=off  N=100  UseFilter=on  TunerSelectOption=Frequency Response Based  InitialConditionSource=internal  InitialConditionForIntegrator=0  InitialConditionForFilter=0  DifferentiatorICPrevScaledInput=0  ExternalReset=none  TrackingMode=off  Kt=1  LimitOutput=off  SatLimitsSource=internal  UpperSaturationLimit=inf  LowerSaturationLimit=-inf  LinearizeAsGain=off  AntiWindupMode=none  Kb=1  LimitIntegrator=off  UpperIntegratorSaturationLimit=inf  LowerIntegratorSaturationLimit=-inf  POutMin=[]  POutMax=[]  IOutMin=[]  IOutMax=[]  DOutMin=[]  DOutMax=[]  NOutMin=[]  NOutMax=[]  SumOutMin=[]  SumOutMax=[]  SaturationOutMin=[]  SaturationOutMax=[]  PParamMin=[]  PParamMax=[]  IParamMin=[]  IParamMax=[]  DParamMin=[]  DParamMax=[]  NParamMin=[]  NParamMax=[]  KbParamMin=[]  KbParamMax=[]  KtParamMin=[]  KtParamMax=[]  KbOutMin=[]  KbOutMax=[]  KtOutMin=[]  KtOutMax=[]  IntegratorOutMin=[]  IntegratorOutMax=[]  FilterOutMin=[]  FilterOutMax=[]  SumI1OutMin=[]  SumI1OutMax=[]  SumI2OutMin=[]  SumI2OutMax=[]  SumI3OutMin=[]  SumI3OutMax=[]  SumI4OutMin=[]  SumI4OutMax=[]  SumDOutMin=[]  SumDOutMax=[]  DifferentiatorOutMin=[]  DifferentiatorOutMax=[]  FilterDiffOutCoefMin=[]  FilterDiffOutCoefMax=[]  ReciprocalOutMin=[]  ReciprocalOutMax=[]  SumDenOutMin=[]  SumDenOutMax=[]  SumNumOutMin=[]  SumNumOutMax=[]  DivideOutMin=[]  DivideOutMax=[]  UdiffTsProdOutMin=[]  UdiffTsProdOutMax=[]  NTsProdOutMin=[]  NTsProdOutMax=[]  UintegralTsProdOutMin=[]  UintegralTsProdOutMax=[]  UngainTsProdOutMin=[]  UngainTsProdOutMax=[]  ClampingZeroOutDataTypeStr=Inherit: Inherit via back propagation  ClampingZeroOutMin=[]  ClampingZeroOutMax=[]  FilterDenConstantOutDataTypeStr=Inherit: Inherit via back propagation  FilterDenConstantOutMin=[]  FilterDenConstantOutMax=[]  PCopyOutDataTypeStr=Inherit: Inherit via back propagation  PCopyOutMin=[]  PCopyOutMax=[]  NCopyOutDataTypeStr=Inherit: Inherit via back propagation  NCopyOutMin=[]  NCopyOutMax=[]  IntegratorContinuousStateAttributes=''  IntegratorStateMustResolveToSignalObject=off  IntegratorRTWStateStorageClass=Auto  FilterContinuousStateAttributes=''  FilterStateMustResolveToSignalObject=off  FilterRTWStateStorageClass=Auto  ParallelPVariant=InternalParameters  IdealPVariant=Disabled  IVariant=InternalParameters  DVariant=InternalParameters  IntegratorVariant=Discrete  SatVariant=Disabled  AWVariant=Passthrough  PCopyVariant=Disabled  TRVariant=Disabled  FdbkBlocksVariant=Forward  IdealPFdbkVariant=Disabled  SatFdbkVariant=Disabled  DerivativeFilterVariant=ForwardEulerFilter  NVariant=InternalParameters  NCopyVariant=Disabled  FilterICVariant=InternalICsFilter  IntegratorICVariant=InternalICs  ExternalResetVariant=Disabled  TRSumVariant=Passthrough  SumFdbkVariant=Disabled  SumVariant=Sum_PID  TsampFilterVariant=InternalTs  TsampNgainVariant=Passthrough  TsampIntegralVariant=Disabled_SignalSpec  ExternalSaturationOutDataTypeStr=Inherit: Same as second input  DerivativeSourceVariant=ErrorSignal  PreIntVariant=InternalPreInt
      settings: LibrarySourceBlock=simulink/Discrete/Discrete PID Controller
  PI_right : slpidlib/PID Controller  Controller=PID  Form=Parallel  TimeDomain=Discrete-time  UseExternalTs=off  SampleTime=0.01  IntegratorMethod=Forward Euler  FilterMethod=Forward Euler  ControllerParametersSource=internal  P=0.02711  I=0.00415  UseKiTs=off  D=0  UseExternalDerivativeSource=off  N=100  UseFilter=on  TunerSelectOption=Transfer Function Based (PID Tuner App)  InitialConditionSource=internal  InitialConditionForIntegrator=0  InitialConditionForFilter=0  DifferentiatorICPrevScaledInput=0  ExternalReset=none  TrackingMode=off  Kt=1  LimitOutput=off  SatLimitsSource=internal  UpperSaturationLimit=inf  LowerSaturationLimit=-inf  LinearizeAsGain=off  AntiWindupMode=none  Kb=1  LimitIntegrator=off  UpperIntegratorSaturationLimit=inf  LowerIntegratorSaturationLimit=-inf  POutMin=[]  POutMax=[]  IOutMin=[]  IOutMax=[]  DOutMin=[]  DOutMax=[]  NOutMin=[]  NOutMax=[]  SumOutMin=[]  SumOutMax=[]  SaturationOutMin=[]  SaturationOutMax=[]  PParamMin=[]  PParamMax=[]  IParamMin=[]  IParamMax=[]  DParamMin=[]  DParamMax=[]  NParamMin=[]  NParamMax=[]  KbParamMin=[]  KbParamMax=[]  KtParamMin=[]  KtParamMax=[]  KbOutMin=[]  KbOutMax=[]  KtOutMin=[]  KtOutMax=[]  IntegratorOutMin=[]  IntegratorOutMax=[]  FilterOutMin=[]  FilterOutMax=[]  SumI1OutMin=[]  SumI1OutMax=[]  SumI2OutMin=[]  SumI2OutMax=[]  SumI3OutMin=[]  SumI3OutMax=[]  SumI4OutMin=[]  SumI4OutMax=[]  SumDOutMin=[]  SumDOutMax=[]  DifferentiatorOutMin=[]  DifferentiatorOutMax=[]  FilterDiffOutCoefMin=[]  FilterDiffOutCoefMax=[]  ReciprocalOutMin=[]  ReciprocalOutMax=[]  SumDenOutMin=[]  SumDenOutMax=[]  SumNumOutMin=[]  SumNumOutMax=[]  DivideOutMin=[]  DivideOutMax=[]  UdiffTsProdOutMin=[]  UdiffTsProdOutMax=[]  NTsProdOutMin=[]  NTsProdOutMax=[]  UintegralTsProdOutMin=[]  UintegralTsProdOutMax=[]  UngainTsProdOutMin=[]  UngainTsProdOutMax=[]  ClampingZeroOutDataTypeStr=Inherit: Inherit via back propagation  ClampingZeroOutMin=[]  ClampingZeroOutMax=[]  FilterDenConstantOutDataTypeStr=Inherit: Inherit via back propagation  FilterDenConstantOutMin=[]  FilterDenConstantOutMax=[]  PCopyOutDataTypeStr=Inherit: Inherit via back propagation  PCopyOutMin=[]  PCopyOutMax=[]  NCopyOutDataTypeStr=Inherit: Inherit via back propagation  NCopyOutMin=[]  NCopyOutMax=[]  IntegratorContinuousStateAttributes=''  IntegratorStateMustResolveToSignalObject=off  IntegratorRTWStateStorageClass=Auto  FilterContinuousStateAttributes=''  FilterStateMustResolveToSignalObject=off  FilterRTWStateStorageClass=Auto  ParallelPVariant=InternalParameters  IdealPVariant=Disabled  IVariant=InternalParameters  DVariant=InternalParameters  IntegratorVariant=Discrete  SatVariant=Disabled  AWVariant=Passthrough  PCopyVariant=Disabled  TRVariant=Disabled  FdbkBlocksVariant=Forward  IdealPFdbkVariant=Disabled  SatFdbkVariant=Disabled  DerivativeFilterVariant=ForwardEulerFilter  NVariant=InternalParameters  NCopyVariant=Disabled  FilterICVariant=InternalICsFilter  IntegratorICVariant=InternalICs  ExternalResetVariant=Disabled  TRSumVariant=Passthrough  SumFdbkVariant=Disabled  SumVariant=Sum_PID  TsampFilterVariant=InternalTs  TsampNgainVariant=Passthrough  TsampIntegralVariant=Disabled_SignalSpec  ExternalSaturationOutDataTypeStr=Inherit: Same as second input  DerivativeSourceVariant=ErrorSignal  PreIntVariant=InternalPreInt
      settings: LibrarySourceBlock=simulink/Discrete/Discrete PID Controller
  RT{,1,3..5,7} (6 alike) : RateTransition  OutPortSampleTime=0.001
  RT2 : RateTransition  OutPortSampleTime=0.01
  RT6 : RateTransition  OutPortSampleTime=0.01
  Sum : Sum  Inputs=|+-
  Sum1 : Sum  Inputs=|+-
  Sum_left_error : Sum  Inputs=|+-
  Sum_right_error : Sum  Inputs=|+-
  u_left_raw : Outport
  u_right_raw : Outport  Port=2
  wires:
  Nbar_right/1 -> Sum1/1
  omega_right_ref/1 -> Sum_right_error/1, Nbar_right/1
  Manual Switch1/1 -> u_left_raw/1
  omega_left_meas/1 -> RT7/1, K_left/1
  K_right/1 -> RT1/1
  K_left/1 -> RT4/1
  Manual Switch/1 -> u_right_raw/1
  omega_left_ref/1 -> Nbar_left/1, Sum_left_error/1
  RT7/1 -> Sum_left_error/2
  omega_right_meas/1 -> RT3/1, K_right/1
  RT3/1 -> Sum_right_error/2
  Sum/1 -> Manual Switch1/2
  Sum_left_error/1 -> RT6/1  "left_error"
  Nbar_left/1 -> Sum/1
  RT4/1 -> Sum/2
  RT1/1 -> Sum1/2
  Sum_right_error/1 -> RT2/1  "right_error"
  RT6/1 -> PI_left/1  "left_error"
  PI_right/1 -> RT/1
  Sum1/1 -> Manual Switch/1
  RT/1 -> Manual Switch/2
  RT2/1 -> PI_right/1  "right_error"
  PI_left/1 -> RT5/1
  RT5/1 -> Manual Switch1/1

== system ME416_Autonomy_Model_Rollback2/HardwareIO/ArmActuators_System ==
  base_servo_cmd : Inport
  femur_servo_cmd : Inport  Port=2
  stepper_enable : Inport  Port=3
  stepper_dir_cmd : Inport  Port=4
  stepper_step_cmd : Inport  Port=5
  gripper_cmd : Inport  Port=6
  "A4988N_Dir " : raspberrypiBasiclib/GPIO Write  Commented=on  BoardProperty=Pi 4 Model B  gpio=22  blockPlatform=Raspberry Pi  PinNumber=17  board=[]  direction=[]
  A4988N_EN : raspberrypiBasiclib/GPIO Write  Commented=on  BoardProperty=Pi 4 Model B  gpio=27  blockPlatform=Raspberry Pi  PinNumber=17  board=[]  direction=[]
  A4988N_Step : raspberrypiBasiclib/PWM  Commented=on  board=Pi 4 Model B  Pin_=17  Frequency=500  blockPlatform=Raspberry Pi
  Base_Servo_PWM : raspberrypiBasiclib/PWM  board=Pi 4 Model B  Pin_=13  Frequency=50  blockPlatform=Raspberry Pi
  Femur_Servo_PWM : raspberrypiBasiclib/GPIO Write  Commented=on  BoardProperty=Pi 4 Model B  gpio=13  blockPlatform=Raspberry Pi  PinNumber=17  board=[]  direction=[]
  Gripper_Servo_PWM : raspberrypiBasiclib/GPIO Write  Commented=on  BoardProperty=Pi 4 Model B  gpio=19  blockPlatform=Raspberry Pi  PinNumber=17  board=[]  direction=[]
  wires:
  femur_servo_cmd/1 -> Femur_Servo_PWM/1
  stepper_dir_cmd/1 -> "A4988N_Dir "/1
  stepper_step_cmd/1 -> A4988N_Step/1
  gripper_cmd/1 -> Gripper_Servo_PWM/1
  stepper_enable/1 -> A4988N_EN/1
  base_servo_cmd/1 -> Base_Servo_PWM/1

== system ME416_Autonomy_Model_Rollback2/HardwareIO/Encoder_System ==
  DriveOutBus : Inport
  Bus Selector : BusSelector  OutputSignals=u_left,u_right,estop_active_out
  L298N_HBridge_Driver : Subsystem
  LeftEncoderQuadrature : Subsystem
  RightEncoderQuadrature : Subsystem
  enc_left_ticks : Outport
  enc_right_ticks : Outport  Port=2
  wires:
  RightEncoderQuadrature/1(enc_right_ticks) -> enc_right_ticks/1  "enc_right_ticks"
  DriveOutBus/1 -> Bus Selector/1
  LeftEncoderQuadrature/1(enc_left_ticks) -> enc_left_ticks/1  "enc_left_ticks"
  Bus Selector/1 -> L298N_HBridge_Driver/1(<u_left>)  "<u_left>"
  Bus Selector/2 -> L298N_HBridge_Driver/2(<u_right>)  "<u_right>"
  Bus Selector/3 -> L298N_HBridge_Driver/3(<estop_active_out>)  "<estop_active_out>"
